simulink model "EMsimulink"  (R2020a)
settings: Solver=VariableStepAuto  StartTime=0.0  StopTime=3  RelTol=1e-3
values from neighbouring files (symbols this model uses):
  b = 3.5E-6    (= 3.5e-06)    [EMscript.m]
  J = 3.22E-6    (= 3.22e-06)    [EMscript.m]
  Kb = 0.03    [EMscript.m]
  Kt = 0.03    [EMscript.m]
  R = 4    [EMscript.m]
  V = 1    [EMscript.m]
settings Model: Creator=diogo  LastModifiedBy=diogo

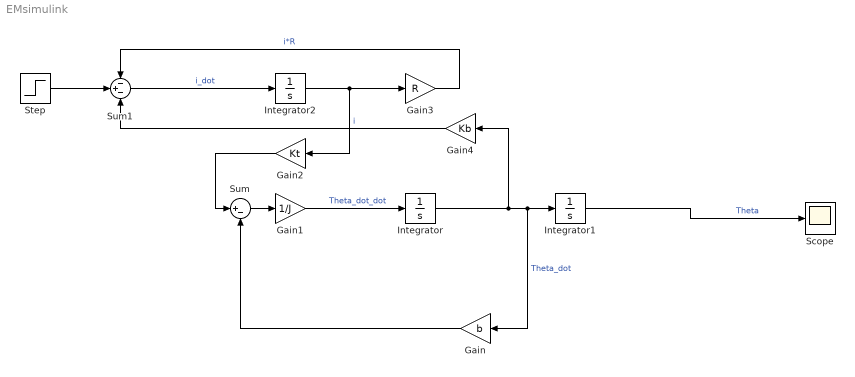
== system EMsimulink ==
  Gain : Gain  Gain=b
  Gain1 : Gain  Gain=1/J
  Gain2 : Gain  Gain=Kt
  Gain3 : Gain  Gain=R
  Gain4 : Gain  Gain=Kb
  Integrator : Integrator
  Integrator1 : Integrator
  Integrator2 : Integrator
  Scope : Scope
  Step : Step  After=V  SampleTime=0
  Sum : Sum  Inputs=|+-
  Sum1 : Sum  Inputs=-+-
  wires:
  Gain1/1 -> Integrator/1  "Theta_dot_dot"
  Integrator/1 -> Gain4/1, Gain/1, Integrator1/1  "Theta_dot"
  Integrator1/1 -> Scope/1  "Theta"
  Step/1 -> Sum1/2
  Sum/1 -> Gain1/1
  Gain/1 -> Sum/2
  Integrator2/1 -> Gain2/1, Gain3/1  "i"
  Sum1/1 -> Integrator2/1  "i_dot"
  Gain2/1 -> Sum/1
  Gain3/1 -> Sum1/1  "i*R"
  Gain4/1 -> Sum1/3
